simulink library "csc_mem_cab_integrated_mems_lib"  (R2014b)
settings: Solver=ode45  StartTime=0.0  StopTime=10.0  RelTol=1e-3
libraries: csc_mum_mems_unit_model_lib x3, util_info_lib x1, util_common_lib x1
settings Model: Creator=escrane  LastModifiedBy=mstewart

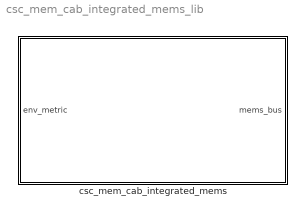
== system csc_mem_cab_integrated_mems_lib ==
  csc_mem_cab_integrated_mems : Subsystem

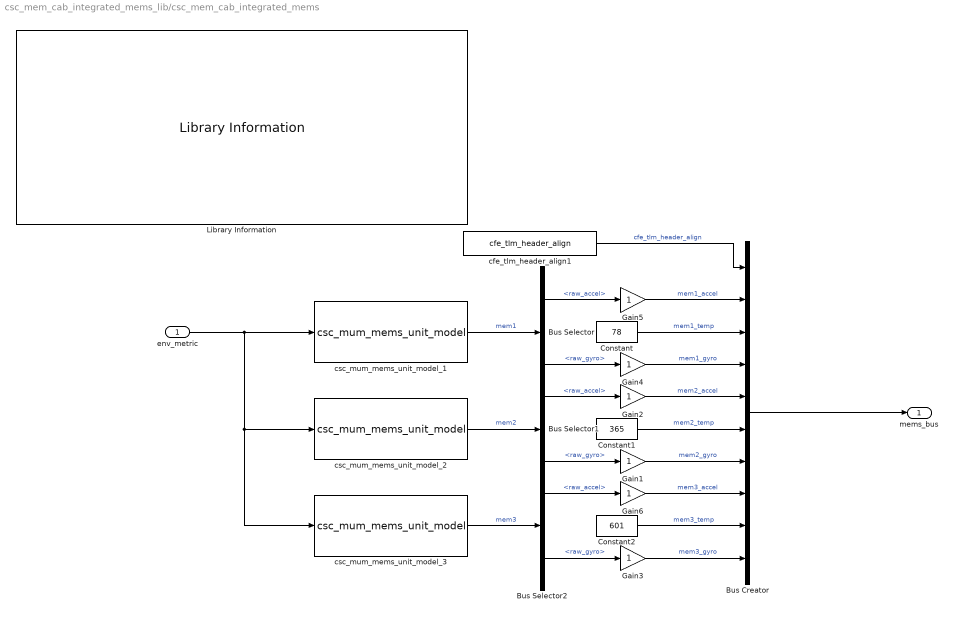
== system csc_mem_cab_integrated_mems_lib/csc_mem_cab_integrated_mems ==
  env_metric : Inport
  Bus Creator : BusCreator  Inputs=10  OutDataTypeStr=Bus: mem_veh_msg  NonVirtualBus=on
  Bus Selector : BusSelector  OutputSignals=raw_accel,raw_gyro
  Bus Selector1 : BusSelector  OutputSignals=raw_accel,raw_gyro
  Bus Selector2 : BusSelector  OutputSignals=raw_accel,raw_gyro
  Constant : Constant  Value=78  OutDataTypeStr=int16
  Constant1 : Constant  Value=365  OutDataTypeStr=int16
  Constant2 : Constant  Value=601  OutDataTypeStr=int16
  Gain{1..6} (6 alike) : Gain  OutDataTypeStr=int16
  Library Information : util_info_lib/Library Information  owner='escrane'
  cfe_tlm_header_align1 : util_common_lib/cfe_tlm_header_align
  csc_mum_mems_unit_model_1 : csc_mum_mems_unit_model_lib/csc_mum_mems_unit_model  my_imu_position=mum1_position  my_imu_dcm=mum1_dcm  my_accel_seed_v=mum1_accel_noise_seed  my_accel_bias_seed_v=mum1_accel_bias_seed  my_gyro_seed_v=mum1_gyro_noise_seed  my_gyro_bias_seed_v=mum1_gyro_bias_seed
  csc_mum_mems_unit_model_2 : csc_mum_mems_unit_model_lib/csc_mum_mems_unit_model  my_imu_position=mum2_position  my_imu_dcm=mum2_dcm  my_accel_seed_v=mum2_accel_noise_seed  my_accel_bias_seed_v=mum2_accel_bias_seed  my_gyro_seed_v=mum2_gyro_noise_seed  my_gyro_bias_seed_v=mum2_gyro_bias_seed
  csc_mum_mems_unit_model_3 : csc_mum_mems_unit_model_lib/csc_mum_mems_unit_model  my_imu_position=mum3_position  my_imu_dcm=mum3_dcm  my_accel_seed_v=mum3_accel_noise_seed  my_accel_bias_seed_v=mum3_accel_bias_seed  my_gyro_seed_v=mum3_gyro_noise_seed  my_gyro_bias_seed_v=mum3_gyro_bias_seed
  mems_bus : Outport
  wires:
  Constant2/1 -> Bus Creator/9  "mem3_temp"
  Constant1/1 -> Bus Creator/6  "mem2_temp"
  Constant/1 -> Bus Creator/3  "mem1_temp"
  cfe_tlm_header_align1/1 -> Bus Creator/1  "cfe_tlm_header_align"
  Gain5/1 -> Bus Creator/2  "mem1_accel"
  Gain4/1 -> Bus Creator/4  "mem1_gyro"
  Gain2/1 -> Bus Creator/5  "mem2_accel"
  Gain1/1 -> Bus Creator/7  "mem2_gyro"
  Gain3/1 -> Bus Creator/10  "mem3_gyro"
  Gain6/1 -> Bus Creator/8  "mem3_accel"
  Bus Selector2/2 -> Gain3/1  "<raw_gyro>"
  Bus Selector2/1 -> Gain6/1  "<raw_accel>"
  Bus Selector1/2 -> Gain1/1  "<raw_gyro>"
  Bus Selector1/1 -> Gain2/1  "<raw_accel>"
  Bus Selector/2 -> Gain4/1  "<raw_gyro>"
  Bus Selector/1 -> Gain5/1  "<raw_accel>"
  csc_mum_mems_unit_model_3/1 -> Bus Selector2/1  "mem3"
  csc_mum_mems_unit_model_2/1 -> Bus Selector1/1  "mem2"
  csc_mum_mems_unit_model_1/1 -> Bus Selector/1  "mem1"
  env_metric/1 -> csc_mum_mems_unit_model_1/1, csc_mum_mems_unit_model_2/1, csc_mum_mems_unit_model_3/1
  Bus Creator/1 -> mems_bus/1
